simulink model "molicel_48v_pack"  (R2026a)
settings: Solver=VariableStepAuto  StopTime=t_stop
values from neighbouring files (symbols this model uses):
  I_load_pack = 18    [molicel_48v_pack_params.m]
  I_pack_max = N_parallel * I_cell_max    (= 180)    [molicel_48v_pack_params.m]
  N_parallel = 4    [molicel_48v_pack_params.m]
  N_series = 13    [molicel_48v_pack_params.m]
  OCV_cell_table = [2.50 2.85 3.16 3.31 3.44 3.52 3.59 3.65 3.74 3.84 3.92 4.02 4.08 4.19]    [molicel_48v_pack_params.m]
  R0_pack = R0_cell * N_series / N_parallel    (= 0.02275)    [molicel_48v_pack_params.m]
  R1_pack = R1_cell * N_series / N_parallel    (= 0.017875)    [molicel_48v_pack_params.m]
  R2_pack = R2_cell * N_series / N_parallel    (= 0.013)    [molicel_48v_pack_params.m]
  SOC_breakpoints = [0 0.02 0.05 0.10 0.20 0.30 0.40 0.50 0.60 0.70 0.80 0.90 0.95 1.00]    [molicel_48v_pack_params.m]
  SOC_initial = 1.0    (= 1)    [molicel_48v_pack_params.m]
  SOC_rate_gain = -1 / (Q_pack_Ah * 3600)    (= -1.54320987654e-05)    [molicel_48v_pack_params.m]
  T_ambient_C = 23    [molicel_48v_pack_params.m]
  T_dis_max_C = 60    [molicel_48v_pack_params.m]
  T_dis_min_C = -40    [molicel_48v_pack_params.m]
  tau1 = 3    [molicel_48v_pack_params.m]
  tau2 = 50    [molicel_48v_pack_params.m]
  V_pack_cutoff = N_series * V_cell_cutoff    (= 32.5)    [molicel_48v_pack_params.m]
libraries: hdlsllib x3
settings Model: Creator=Razvan  LastModifiedBy=Razvan

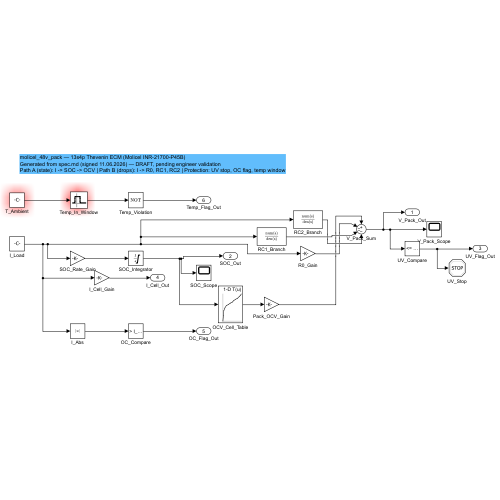
[thumbnail: Simulink's stored preview of the top-level diagram]
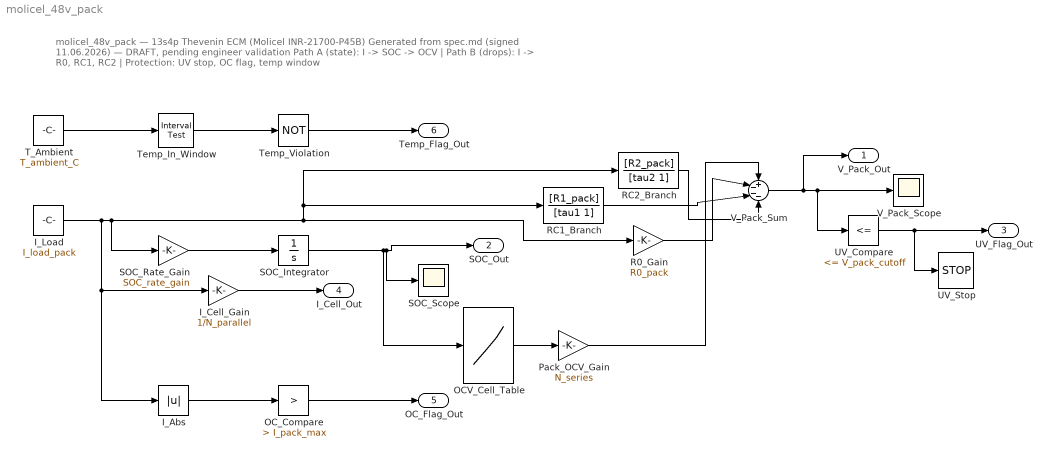
== system molicel_48v_pack ==
  note: molicel_48v_pack — 13s4p Thevenin ECM (Molicel INR-21700-P45B)
      | Generated from spec.md (signed 11.06.2026) — DRAFT, pending engineer validation
      | Path A (state): I -> SOC -> OCV | Path B (drops): I -> R0, RC1, RC2 | Protection: UV stop, OC flag, temp window
  I_Abs : Abs  Description=spec §5: |I_pack| for overcurrent check
  I_Cell_Gain : Gain  Description=spec §4: per-cell current = pack current / 4 (perfect sharing assumption)  Gain=1/N_parallel
  I_Load : Constant  Description=spec §6: constant discharge 18 A (1C pack rate). Variable: I_load_pack  Value=I_load_pack
  OCV_Cell_Table : Lookup_n-D  Description=spec §3: OCV(SOC) table, test report p.7 0.2C curve (graphical read)  NumberOfTableDimensions=1  BreakpointsForDimension1=SOC_breakpoints  Table=OCV_cell_table
  OC_Compare : hdlsllib/Logic and Bit Operations/Compare To Constant  Description=spec §5: overcurrent flag, |I_pack| > 180 A (4 x 45 A DS limit)  relop=>  const=I_pack_max  OutDataTypeStr=boolean
  Pack_OCV_Gain : Gain  Description=spec §4: 13 cells in series -> pack OCV = 13 x cell OCV  Gain=N_series
  R0_Gain : Gain  Description=spec §4: Pack R0 = 7 mOhm x 13/4 = 22.75 mOhm (cell R0 from DS AC impedance)  Gain=R0_pack
  RC1_Branch : TransferFcn  Description=spec §3/§4: fast RC branch, R1_pack=17.875 mOhm, tau1=3 s (ASSUMED, anchored to DS 15 mOhm @10s)  Numerator=[R1_pack]  Denominator=[tau1 1]
  RC2_Branch : TransferFcn  Description=spec §3/§4: slow RC branch, R2_pack=13.0 mOhm, tau2=50 s (ASSUMED)  Numerator=[R2_pack]  Denominator=[tau2 1]
  SOC_Integrator : Integrator  Description=spec §6: IC = 100% SOC; saturated [0,1] (nonphysical SOC guard)  InitialCondition=SOC_initial  LimitOutput=on  UpperSaturationLimit=1  LowerSaturationLimit=0
  SOC_Rate_Gain : Gain  Description=spec §4: SOC rate gain = -1/(18 Ah * 3600) = -1.5432e-5 1/(s*A)  Gain=SOC_rate_gain
  SOC_Scope : Scope
  T_Ambient : Constant  Description=spec §6: scenario ambient 23 degC (TR test conditions)  Value=T_ambient_C
  Temp_In_Window : hdlsllib/Logic and Bit Operations/Interval Test  Description=spec §5: discharge temp window -40..+60 degC (DS)  IntervalClosedRight=on  uplimit=T_dis_max_C  IntervalClosedLeft=on  lowlimit=T_dis_min_C  OutDataTypeStr=boolean
  Temp_Violation : Logic  Description=spec §5: flag = NOT(in window)  Operator=NOT  AllPortsSameDT=off  OutDataTypeStr=boolean
  UV_Compare : hdlsllib/Logic and Bit Operations/Compare To Constant  Description=spec §5: undervoltage cutoff, pack < 32.5 V (13 x 2.5 V DS cutoff)  relop=<=  const=V_pack_cutoff  OutDataTypeStr=boolean
  UV_Stop : Stop  Description=spec §6: stop condition - discharge terminated at pack UV cutoff
  V_Pack_Scope : Scope
  V_Pack_Sum : Sum  Description=spec §3: V_pack = OCV_pack - V_R0 - V_RC1 - V_RC2  Inputs=+---
  V_Pack_Out : Outport  Description=Pack terminal voltage [V] -> out.yout{1}
  SOC_Out : Outport  Description=Pack SOC [-] -> out.yout{2}  Port=2
  UV_Flag_Out : Outport  Description=Undervoltage flag [bool]  Port=3
  I_Cell_Out : Outport  Description=Per-cell current [A], must stay <= 45 A (DS limit, AC5)  Port=4
  OC_Flag_Out : Outport  Description=Overcurrent flag [bool]  Port=5
  Temp_Flag_Out : Outport  Description=Temperature window violation flag [bool]  Port=6
  wires:
  V_Pack_Sum/1 -> UV_Compare/1, V_Pack_Scope/1, V_Pack_Out/1
  RC2_Branch/1 -> V_Pack_Sum/4
  RC1_Branch/1 -> V_Pack_Sum/3
  R0_Gain/1 -> V_Pack_Sum/2
  Pack_OCV_Gain/1 -> V_Pack_Sum/1
  OCV_Cell_Table/1 -> Pack_OCV_Gain/1
  SOC_Integrator/1 -> SOC_Scope/1, SOC_Out/1, OCV_Cell_Table/1
  SOC_Rate_Gain/1 -> SOC_Integrator/1
  I_Load/1 -> I_Abs/1, I_Cell_Gain/1, RC1_Branch/1, RC2_Branch/1, R0_Gain/1, SOC_Rate_Gain/1
  UV_Compare/1 -> UV_Flag_Out/1, UV_Stop/1
  I_Cell_Gain/1 -> I_Cell_Out/1
  I_Abs/1 -> OC_Compare/1
  OC_Compare/1 -> OC_Flag_Out/1
  T_Ambient/1 -> Temp_In_Window/1
  Temp_In_Window/1 -> Temp_Violation/1
  Temp_Violation/1 -> Temp_Flag_Out/1
